simulink model "rolingroad[Conflict]"  (R2015a)
settings: Solver=ode45  StartTime=0.0  StopTime=10.0  RelTol=1e-3
libraries: simulink x1
settings Model: Creator=jonathan  LastModifiedBy=jonathan

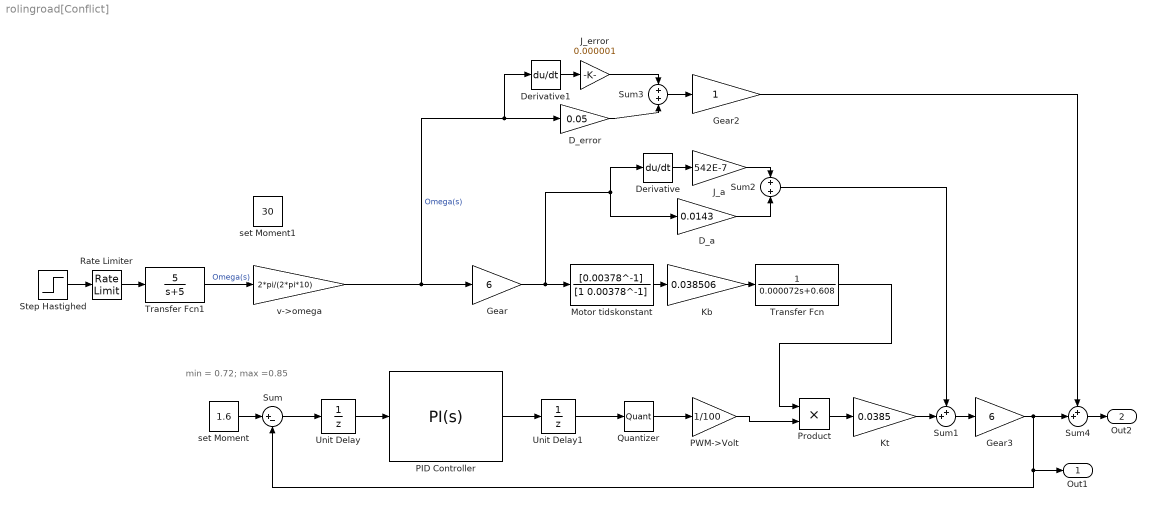
== system rolingroad[Conflict] ==
  note: min = 0.72; max =0.85
  D_a : Gain  Gain=0.0143
  D_error : Gain  Gain=0.05
  Derivative : Derivative  CoefficientInTFapproximation=1000000
  Derivative1 : Derivative  CoefficientInTFapproximation=1000000
  Gear : Gain  Gain=6
  Gear2 : Gain
  Gear3 : Gain  Gain=6
  J_a : Gain  Gain=542E-7
  J_error : Gain  Gain=0.000001
  Kb : Gain  Gain=0.038506
  Kt : Gain  Gain=0.0385
  Motor tidskonstant : TransferFcn  Numerator=[0.00378^-1]  Denominator=[1 0.00378^-1]
  PID Controller : simulink/Continuous/PID Controller  Controller=PI  TimeDomain=Continuous-time  SampleTime=-1  IntegratorMethod=Forward Euler  FilterMethod=Forward Euler  Form=Parallel  UseFilter=off  ControllerParametersSource=internal  P=5  I=6000  D=0  N=100  InitialConditionSource=internal  InitialConditionForIntegrator=0  InitialConditionForFilter=0  ExternalReset=none  LimitOutput=on  UpperSaturationLimit=100  LowerSaturationLimit=0  LinearizeAsGain=off  AntiWindupMode=clamping  Kb=1  TrackingMode=off  Kt=1  PParamMin=[]  PParamMax=[]  IParamMin=[]  IParamMax=[]  DParamMin=[]  DParamMax=[]  NParamMin=[]  NParamMax=[]  KbParamMin=[]  KbParamMax=[]  KtParamMin=[]  KtParamMax=[]  POutMin=[]  POutMax=[]  IOutMin=[]  IOutMax=[]  DOutMin=[]  DOutMax=[]  NOutMin=[]  NOutMax=[]  KbOutMin=[]  KbOutMax=[]  KtOutMin=[]  KtOutMax=[]  IntegratorOutMin=[]  IntegratorOutMax=[]  FilterOutMin=[]  FilterOutMax=[]  SumOutMin=[]  SumOutMax=[]  SumI1OutMin=[]  SumI1OutMax=[]  SumI2OutMin=[]  SumI2OutMax=[]  SumI3OutMin=[]  SumI3OutMax=[]  SumDOutMin=[]  SumDOutMax=[]  SaturationOutMin=[]  SaturationOutMax=[]  IntegratorContinuousStateAttributes=''  IntegratorStateMustResolveToSignalObject=off  IntegratorRTWStateStorageClass=Auto  FilterContinuousStateAttributes=''  FilterStateMustResolveToSignalObject=off  FilterRTWStateStorageClass=Auto  DifferentiatorICPrevScaledInput=0  DifferentiatorOutMin=[]  DifferentiatorOutMax=[]
  PWM->Volt : Gain  Gain=1/100
  Product : Product
  Quantizer : Quantizer
  Rate Limiter : RateLimiter  RisingSlewLimit=5
  Step Hastighed : Step  After=30  SampleTime=0
  Sum : Sum  Inputs=|+-
  Sum1 : Sum  Inputs=++|
  Sum2 : Sum  Inputs=+|+
  Sum3 : Sum  Inputs=+|+
  Sum4 : Sum  Inputs=++|
  Transfer Fcn : TransferFcn  Denominator=[0.000072 0.608]
  Transfer Fcn1 : TransferFcn  Numerator=[5]  Denominator=[1 5]
  Unit Delay : UnitDelay  SampleTime=0.005
  Unit Delay1 : UnitDelay  SampleTime=0.005
  set Moment : Constant  Value=1.6
  set Moment1 : Constant  Value=30
  v->omega : Gain  Gain=2*pi/(2*pi*10)
  Out1 : Outport
  Out2 : Outport  Port=2
  wires:
  set Moment/1 -> Sum/1
  Kb/1 -> Transfer Fcn/1
  PWM->Volt/1 -> Product/2
  Product/1 -> Kt/1
  Quantizer/1 -> PWM->Volt/1
  Derivative/1 -> J_a/1
  D_a/1 -> Sum2/2
  J_a/1 -> Sum2/1
  v->omega/1 -> Derivative1/1, D_error/1, Gear/1  "Omega(s)"
  Derivative1/1 -> J_error/1
  D_error/1 -> Sum3/2
  J_error/1 -> Sum3/1
  Sum3/1 -> Gear2/1
  Sum2/1 -> Sum1/1
  Sum1/1 -> Gear3/1
  Gear2/1 -> Sum4/1
  Sum4/1 -> Out2/1
  Step Hastighed/1 -> Rate Limiter/1
  Rate Limiter/1 -> Transfer Fcn1/1
  Sum/1 -> Unit Delay/1
  Unit Delay/1 -> PID Controller/1
  Unit Delay1/1 -> Quantizer/1
  PID Controller/1 -> Unit Delay1/1
  Transfer Fcn1/1 -> v->omega/1  "Omega(s)"
  Transfer Fcn/1 -> Product/1
  Motor tidskonstant/1 -> Kb/1
  Gear/1 -> D_a/1, Derivative/1, Motor tidskonstant/1
  Kt/1 -> Sum1/2
  Gear3/1 -> Sum4/2, Out1/1, Sum/2
